simulink model "mpc_track_sim"  (R2014b)
settings: Solver=ode3  StartTime=0.0  StopTime=100.0  FixedStep=0.01  RelTol=1e-3
values from neighbouring files (symbols this model uses):
  h = 1/100    (= 0.01)    [PlantModelQuadSimpleLinear.m]
  sys_d = c2d(sys_c,h)    [PlantModelQuadSimpleLinear.m]
settings Model: Creator=mlab-retro  LastModifiedBy=mlab-retro

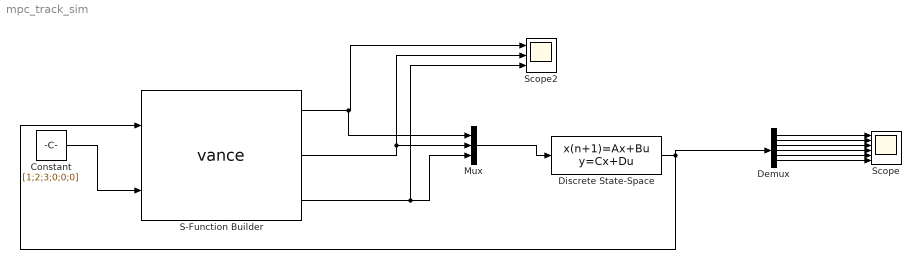
== system mpc_track_sim ==
  Constant : Constant  Value=[1;2;3;0;0;0]
  Demux : Demux  Outputs=6
  Discrete State-Space : DiscreteStateSpace  A=sys_d.a  B=sys_d.b  C=sys_d.c  D=sys_d.d  X0=[0;0;0;0;0;0];  SampleTime=h
  Mux : Mux  Inputs=3
  S-Function Builder : S-Function  InitFcn=try, set_param(gcb,'FunctionName','vance'), end  FunctionName=vance  SFunctionModules=vance_wrapper ldl matrix_support solver util  EnableBusSupport=off  mask(S-Function Builder){}
      mask help: Simulink:masks:SFunctionBuilder_MD
      mask init:
      | val = [[.9  0.75 0.75 1 1 .9 .9 1]',[1 1 0.75 0.75 .9 .9 1 .9]'];try , sys = get_param(gcb,'SfunBuilderFcnName');if isempty(sys), sys = get_param(gcb,'FunctionName'); end,catch, sys = get_param(gcb,'FunctionName'); end
      settings: CopyFcn=set_param(gcbh,'LinkStatus','none')  PreSaveFcn=try, set_param(gcb,'FunctionName','vance'), end  OpenFcn=sfunctionwizard(gcbh)
      mask Display: plot(val(:,1),val(:,2)),disp(sys), port_label('input',1,'x_hat'), port_label('input',2,'x_ref'), port_label('output',1,'theta'), port_label('output',2,'phi'), port_label('output',3,'thrust')
  Scope : Scope  NumInputPorts=6
      settings: TimeRange=100  YMin=-10~-10~-10~-10~-10~-20  YMax=10~10~10~10~10~20
  Scope2 : Scope  NumInputPorts=3
      settings: TimeRange=49.99  YMin=-2e-16~-2e-17~-1e-12  YMax=4e-16~2e-17~5.000000000000001e-13  SaveName=ScopeData2  SampleInput=on
  wires:
  S-Function Builder/1 -> Mux/1, Scope2/1
  Mux/1 -> Discrete State-Space/1
  S-Function Builder/2 -> Mux/2, Scope2/2
  S-Function Builder/3 -> Scope2/3, Mux/3
  Demux/2 -> Scope/2
  Demux/4 -> Scope/4
  Demux/1 -> Scope/1
  Demux/3 -> Scope/3
  Demux/5 -> Scope/5
  Demux/6 -> Scope/6
  Discrete State-Space/1 -> S-Function Builder/1, Demux/1
  Constant/1 -> S-Function Builder/2
